simulink model "DCMG_6unit"  (R2018a)
settings: Solver=VariableStepAuto  StartTime=0.0  StopTime=3  FixedStep=0.1e-3  RelTol=1e-3
undefined symbols (not defined in the file): ALPHA, g12, g14, g23, g24, g36, g45, g56, k_ii_1, k_ii_2, k_ii_3, k_ii_4, k_ii_5, k_ii_6, k_iv_1, k_iv_2, k_iv_3, k_iv_4, k_iv_5, k_iv_6, k_pi_1, k_pi_2, k_pi_3, k_pi_4, k_pi_5, k_pi_6, k_pv_1, k_pv_2, k_pv_3, k_pv_4, k_pv_5, k_pv_6, n, p_fraction, p_k_sup, P_load_inf, P_load_sup, p_stairs, rd1, rd2, rd3, rd4, rd5, rd6, rs1, rs2, rs3, rs4, rs5, rs6, tau, time1, time2, time3, V_ref, Zout_den_source, Zout_num_source
libraries: fl_lib x62, nesl_utility x44, elec_lib x12, simulink x2
settings Model: Creator=Marco  LastModifiedBy=carna

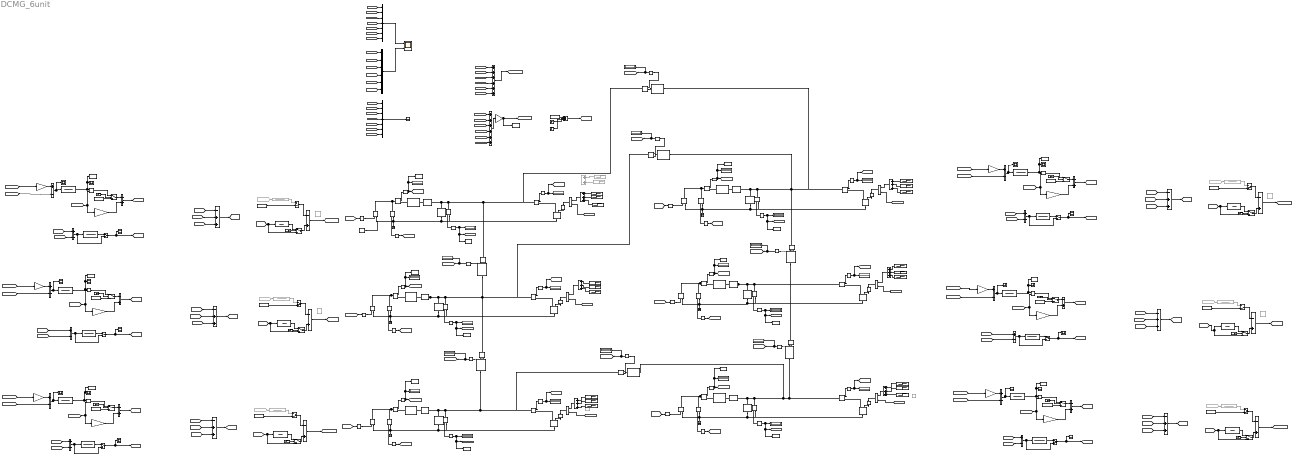
== system DCMG_6unit ==
  note: DELTA I
  note: Delta v 3
  note: I MG
  note: Delta v 1
  note: Delta R droop
  note: V MG
  note: DELTA I
  note: Delta R droop
  note: DELTA I
  note: Delta R droop
  note: Delta v 2
  note: Delta R droop
  note: Delta v 2
  note: DELTA I
  note: Delta R droop
  note: Delta R droop
  note: DELTA I
  note: Delta v 3
  note: Delta v 1
  note: DELTA I
  Add{1..2,5,7,10,12,22..23,25,31,36,38} (12 alike) : Sum  Inputs=+-
  Add{4,6,9,11,13,17,24,26,28,35,37,40} (12 alike) : Sum  Inputs=-+
  Add{3,8,14,27,34,39} (6 alike) : Sum  Inputs=-++
  Add15 : Sum  Inputs=++++++
  Add16 : Sum  Inputs=++++++
  Add{18,20..21,29,32..33,46} (7 alike) : Sum  Inputs=+++
  Add19 : Sum  Commented=on
  C bus 1 : elec_lib/Passive Devices/Capacitor  enable_table=0  c=C1 F  Cvec=[1.0e-5, 1.0e-6] F  Vvec=[0.0, 10.0] V  CV_table_symmetry=1  C_tol=5  enable_C_tol=0  tol_distribution=1  nSigma=4  r=1e-6 Ohm  g=0 1/Ohm  enable_operating_limits=0  operating_limit_action=2  max_working_voltage_range=[-25.0, 25.0] V  power_rating=1 W  enable_faults=0  fault_action=1  Cscale_faulted=100  R_faulted=1e-3 Ohm  G_faulted=0 1/Ohm  tau_fault=1e-3 s  enable_temporal_fault=0  t_fault=1 s  enable_behavioral_fault=0  max_permissible_voltage_range=[-100.0, 100.0] V  t_fail_on_voltage=1 s  i_specify=off  i_priority=None  i=0 A  i_nominal_specify=off  i_nominal_unit=A  i_nominal_value=1  v_specify=off  v_priority=None  v=0 V  v_nominal_specify=off  v_nominal_unit=V  v_nominal_value=1  vc_specify=off  vc_priority=High  vc=0 V  vc_nominal_specify=off  vc_nominal_unit=V  vc_nominal_value=1
  C bus 2 : elec_lib/Passive Devices/Capacitor  enable_table=0  c=C2 F  Cvec=[1.0e-5, 1.0e-6] F  Vvec=[0.0, 10.0] V  CV_table_symmetry=1  C_tol=5  enable_C_tol=0  tol_distribution=1  nSigma=4  r=1e-6 Ohm  g=0 1/Ohm  enable_operating_limits=0  operating_limit_action=2  max_working_voltage_range=[-25.0, 25.0] V  power_rating=1 W  enable_faults=0  fault_action=1  Cscale_faulted=100  R_faulted=1e-3 Ohm  G_faulted=0 1/Ohm  tau_fault=1e-3 s  enable_temporal_fault=0  t_fault=1 s  enable_behavioral_fault=0  max_permissible_voltage_range=[-100.0, 100.0] V  t_fail_on_voltage=1 s  i_specify=off  i_priority=None  i=0 A  i_nominal_specify=off  i_nominal_unit=A  i_nominal_value=1  v_specify=off  v_priority=None  v=0 V  v_nominal_specify=off  v_nominal_unit=V  v_nominal_value=1  vc_specify=off  vc_priority=High  vc=0 V  vc_nominal_specify=off  vc_nominal_unit=V  vc_nominal_value=1
  C bus 3 : elec_lib/Passive Devices/Capacitor  enable_table=0  c=C3 F  Cvec=[1.0e-5, 1.0e-6] F  Vvec=[0.0, 10.0] V  CV_table_symmetry=1  C_tol=5  enable_C_tol=0  tol_distribution=1  nSigma=4  r=1e-6 Ohm  g=0 1/Ohm  enable_operating_limits=0  operating_limit_action=2  max_working_voltage_range=[-25.0, 25.0] V  power_rating=1 W  enable_faults=0  fault_action=1  Cscale_faulted=100  R_faulted=1e-3 Ohm  G_faulted=0 1/Ohm  tau_fault=1e-3 s  enable_temporal_fault=0  t_fault=1 s  enable_behavioral_fault=0  max_permissible_voltage_range=[-100.0, 100.0] V  t_fail_on_voltage=1 s  i_specify=off  i_priority=None  i=0 A  i_nominal_specify=off  i_nominal_unit=A  i_nominal_value=1  v_specify=off  v_priority=None  v=0 V  v_nominal_specify=off  v_nominal_unit=V  v_nominal_value=1  vc_specify=off  vc_priority=High  vc=0 V  vc_nominal_specify=off  vc_nominal_unit=V  vc_nominal_value=1
  C bus 4 : elec_lib/Passive Devices/Capacitor  enable_table=0  c=C4 F  Cvec=[1.0e-5, 1.0e-6] F  Vvec=[0.0, 10.0] V  CV_table_symmetry=1  C_tol=5  enable_C_tol=0  tol_distribution=1  nSigma=4  r=1e-6 Ohm  g=0 1/Ohm  enable_operating_limits=0  operating_limit_action=2  max_working_voltage_range=[-25.0, 25.0] V  power_rating=1 W  enable_faults=0  fault_action=1  Cscale_faulted=100  R_faulted=1e-3 Ohm  G_faulted=0 1/Ohm  tau_fault=1e-3 s  enable_temporal_fault=0  t_fault=1 s  enable_behavioral_fault=0  max_permissible_voltage_range=[-100.0, 100.0] V  t_fail_on_voltage=1 s  i_specify=off  i_priority=None  i=0 A  i_nominal_specify=off  i_nominal_unit=A  i_nominal_value=1  v_specify=off  v_priority=None  v=0 V  v_nominal_specify=off  v_nominal_unit=V  v_nominal_value=1  vc_specify=off  vc_priority=High  vc=0 V  vc_nominal_specify=off  vc_nominal_unit=V  vc_nominal_value=1
  C bus 5 : elec_lib/Passive Devices/Capacitor  enable_table=0  c=C5 F  Cvec=[1.0e-5, 1.0e-6] F  Vvec=[0.0, 10.0] V  CV_table_symmetry=1  C_tol=5  enable_C_tol=0  tol_distribution=1  nSigma=4  r=1e-6 Ohm  g=0 1/Ohm  enable_operating_limits=0  operating_limit_action=2  max_working_voltage_range=[-25.0, 25.0] V  power_rating=1 W  enable_faults=0  fault_action=1  Cscale_faulted=100  R_faulted=1e-3 Ohm  G_faulted=0 1/Ohm  tau_fault=1e-3 s  enable_temporal_fault=0  t_fault=1 s  enable_behavioral_fault=0  max_permissible_voltage_range=[-100.0, 100.0] V  t_fail_on_voltage=1 s  i_specify=off  i_priority=None  i=0 A  i_nominal_specify=off  i_nominal_unit=A  i_nominal_value=1  v_specify=off  v_priority=None  v=0 V  v_nominal_specify=off  v_nominal_unit=V  v_nominal_value=1  vc_specify=off  vc_priority=High  vc=0 V  vc_nominal_specify=off  vc_nominal_unit=V  vc_nominal_value=1
  C bus 6 : elec_lib/Passive Devices/Capacitor  enable_table=0  c=C6 F  Cvec=[1.0e-5, 1.0e-6] F  Vvec=[0.0, 10.0] V  CV_table_symmetry=1  C_tol=5  enable_C_tol=0  tol_distribution=1  nSigma=4  r=1e-6 Ohm  g=0 1/Ohm  enable_operating_limits=0  operating_limit_action=2  max_working_voltage_range=[-25.0, 25.0] V  power_rating=1 W  enable_faults=0  fault_action=1  Cscale_faulted=100  R_faulted=1e-3 Ohm  G_faulted=0 1/Ohm  tau_fault=1e-3 s  enable_temporal_fault=0  t_fault=1 s  enable_behavioral_fault=0  max_permissible_voltage_range=[-100.0, 100.0] V  t_fail_on_voltage=1 s  i_specify=off  i_priority=None  i=0 A  i_nominal_specify=off  i_nominal_unit=A  i_nominal_value=1  v_specify=off  v_priority=None  v=0 V  v_nominal_specify=off  v_nominal_unit=V  v_nominal_value=1  vc_specify=off  vc_priority=High  vc=0 V  vc_nominal_specify=off  vc_nominal_unit=V  vc_nominal_value=1
  Close loop equivalent1 : TransferFcn  Numerator=[k_pv_1 k_iv_1 ]  Denominator=[1 0]
  Close loop equivalent{2,9..12,18} (6 alike) : TransferFcn  Numerator=[1 ]  Denominator=[tau 1]
  Close loop equivalent13 : TransferFcn  Numerator=[k_pv_5 k_iv_5 ]  Denominator=[1 0]
  Close loop equivalent{4,6,8,14..15,17} (6 alike) : TransferFcn  Commented=on  Numerator=Zout_num_source  Denominator=Zout_den_source
  Close loop equivalent16 : TransferFcn  Numerator=[k_pv_6 k_iv_6 ]  Denominator=[1 0]
  Close loop equivalent3 : TransferFcn  Numerator=[k_pv_2 k_iv_2 ]  Denominator=[1 0]
  Close loop equivalent5 : TransferFcn  Numerator=[k_pv_4 k_iv_4 ]  Denominator=[1 0]
  Close loop equivalent7 : TransferFcn  Numerator=[k_pv_3 k_iv_3 ]  Denominator=[1 0]
  Constant{1..3,5..10,15..16,18} (12 alike) : Constant  Value=0
  Constant4 : Constant  Value=V_ref
  Controlled Current Source{1..3,5..7} (6 alike) : fl_lib/Electrical/Electrical Sources/Controlled Current Source
  Controlled Voltage Source{,1..5} (6 alike) : fl_lib/Electrical/Electrical Sources/Controlled Voltage Source
  Current cloop transfer- Transport Delay{1..4} (4 alike) : TransportDelay  Commented=on  DelayTime=0.1e-3
  Current load {1..6} (6 alike) : fl_lib/Electrical/Electrical Sensors/Current Sensor
  Current output {1..13} (13 alike) : fl_lib/Electrical/Electrical Sensors/Current Sensor
  Display{,1..24} (25 alike) : Display
  Divide{1..6} (6 alike) : Product  Inputs=*/
  Electrical Reference{,1..5} (6 alike) : fl_lib/Electrical/Electrical Elements/Electrical Reference
  From17 : From  Commented=on  GotoTag=io_source_2
  From26 : From  Commented=on  GotoTag=io_source_1
  From29 : From  Commented=on  GotoTag=io_source_3
  From56 : From  Commented=on  GotoTag=io_source_2
  From63 : From  Commented=on  GotoTag=io_source_1
  From65 : From  Commented=on  GotoTag=io_source_3
  Gain1 : Gain  Gain=ALPHA(1,1)
  Gain10 : Gain  Gain=ALPHA(5,5)
  Gain11 : Gain  Gain=rd5
  Gain12 : Gain  Gain=ALPHA(6,6)
  Gain13 : Gain  Gain=rd6
  Gain2 : Gain  Gain=rd1
  Gain3 : Gain  Gain=ALPHA(2,2)
  Gain4 : Gain  Gain=rd2
  Gain5 : Gain  Gain=1/n
  Gain6 : Gain  Gain=ALPHA(3,3)
  Gain7 : Gain  Gain=rd3
  Gain8 : Gain  Gain=ALPHA(4,4)
  Gain9 : Gain  Gain=rd4
  L serie 1 : elec_lib/Passive Devices/Inductor  l=L1 H  L_tol=5  enable_L_tol=0  tol_distribution=1  nSigma=4  r=0 Ohm  g=1e-9 1/Ohm  enable_operating_limits=0  operating_limit_action=2  max_working_current=1 A  power_rating=1 W  enable_faults=0  fault_action=1  lambdaPercent=50  k_faulted=0.9999  turnsShort=0  openCct=0  groundShort=0  groundShortG=0 1/Ohm  tau_fault=1e-3 s  enable_temporal_fault=0  t_fault=1 s  enable_behavioral_fault=0  max_permissible_voltage=100 V  n_fail_on_voltage=1  max_permissible_current=1 A  t_fail_on_current=1 s  i_L_specify=off  i_L_priority=High  i_L=0 A  i_L_nominal_specify=off  i_L_nominal_unit=A  i_L_nominal_value=1
      settings: SourceProductName=Simscape Electronics  SourceProductBaseCode=SN
  L serie 2 : elec_lib/Passive Devices/Inductor  l=L2 H  L_tol=20  enable_L_tol=0  tol_distribution=1  nSigma=4  r=0 Ohm  g=1e-9 1/Ohm  enable_operating_limits=0  operating_limit_action=2  max_working_current=1 A  power_rating=1 W  enable_faults=0  fault_action=1  lambdaPercent=50  k_faulted=0.9999  turnsShort=0  openCct=0  groundShort=0  groundShortG=0 1/Ohm  tau_fault=1e-3 s  enable_temporal_fault=0  t_fault=1 s  enable_behavioral_fault=0  max_permissible_voltage=100 V  n_fail_on_voltage=1  max_permissible_current=1 A  t_fail_on_current=1 s  i_L_specify=off  i_L_priority=High  i_L=0 A  i_L_nominal_specify=off  i_L_nominal_unit=A  i_L_nominal_value=1
      settings: SourceProductName=Simscape Electronics  SourceProductBaseCode=SN
  L serie 3 : elec_lib/Passive Devices/Inductor  l=L3 H  L_tol=20  enable_L_tol=0  tol_distribution=1  nSigma=4  r=0 Ohm  g=1e-9 1/Ohm  enable_operating_limits=0  operating_limit_action=2  max_working_current=1 A  power_rating=1 W  enable_faults=0  fault_action=1  lambdaPercent=50  k_faulted=0.9999  turnsShort=0  openCct=0  groundShort=0  groundShortG=0 1/Ohm  tau_fault=1e-3 s  enable_temporal_fault=0  t_fault=1 s  enable_behavioral_fault=0  max_permissible_voltage=100 V  n_fail_on_voltage=1  max_permissible_current=1 A  t_fail_on_current=1 s  i_L_specify=off  i_L_priority=High  i_L=0 A  i_L_nominal_specify=off  i_L_nominal_unit=A  i_L_nominal_value=1
      settings: SourceProductName=Simscape Electronics  SourceProductBaseCode=SN
  L serie 4 : elec_lib/Passive Devices/Inductor  l=L4 H  L_tol=20  enable_L_tol=0  tol_distribution=1  nSigma=4  r=0 Ohm  g=1e-9 1/Ohm  enable_operating_limits=0  operating_limit_action=2  max_working_current=1 A  power_rating=1 W  enable_faults=0  fault_action=1  lambdaPercent=50  k_faulted=0.9999  turnsShort=0  openCct=0  groundShort=0  groundShortG=0 1/Ohm  tau_fault=1e-3 s  enable_temporal_fault=0  t_fault=1 s  enable_behavioral_fault=0  max_permissible_voltage=100 V  n_fail_on_voltage=1  max_permissible_current=1 A  t_fail_on_current=1 s  i_L_specify=off  i_L_priority=High  i_L=0 A  i_L_nominal_specify=off  i_L_nominal_unit=A  i_L_nominal_value=1
      settings: SourceProductName=Simscape Electronics  SourceProductBaseCode=SN
  L serie 5 : elec_lib/Passive Devices/Inductor  l=L5 H  L_tol=20  enable_L_tol=0  tol_distribution=1  nSigma=4  r=0 Ohm  g=1e-9 1/Ohm  enable_operating_limits=0  operating_limit_action=2  max_working_current=1 A  power_rating=1 W  enable_faults=0  fault_action=1  lambdaPercent=50  k_faulted=0.9999  turnsShort=0  openCct=0  groundShort=0  groundShortG=0 1/Ohm  tau_fault=1e-3 s  enable_temporal_fault=0  t_fault=1 s  enable_behavioral_fault=0  max_permissible_voltage=100 V  n_fail_on_voltage=1  max_permissible_current=1 A  t_fail_on_current=1 s  i_L_specify=off  i_L_priority=High  i_L=0 A  i_L_nominal_specify=off  i_L_nominal_unit=A  i_L_nominal_value=1
      settings: SourceProductName=Simscape Electronics  SourceProductBaseCode=SN
  L serie 6 : elec_lib/Passive Devices/Inductor  l=L6 H  L_tol=20  enable_L_tol=0  tol_distribution=1  nSigma=4  r=0 Ohm  g=1e-9 1/Ohm  enable_operating_limits=0  operating_limit_action=2  max_working_current=1 A  power_rating=1 W  enable_faults=0  fault_action=1  lambdaPercent=50  k_faulted=0.9999  turnsShort=0  openCct=0  groundShort=0  groundShortG=0 1/Ohm  tau_fault=1e-3 s  enable_temporal_fault=0  t_fault=1 s  enable_behavioral_fault=0  max_permissible_voltage=100 V  n_fail_on_voltage=1  max_permissible_current=1 A  t_fail_on_current=1 s  i_L_specify=off  i_L_priority=High  i_L=0 A  i_L_nominal_specify=off  i_L_nominal_unit=A  i_L_nominal_value=1
      settings: SourceProductName=Simscape Electronics  SourceProductBaseCode=SN
  Manual Switch{1,3,5,7,9,12} (6 alike) : ManualSwitch
  Manual Switch{2,4,6,8,10..11} (6 alike) : ManualSwitch  CurrentSetting=0
  Mux : Mux  Inputs=6
  Mux1 : Mux  Inputs=7
  Mux2 : Mux  Inputs=7
  PI i : TransferFcn  Numerator=[k_pi_1 k_ii_1 ]  Denominator=[1 0]
  PI i 1 : TransferFcn  Numerator=[k_pi_5 k_ii_5 ]  Denominator=[1 0]
  PI i 2 : TransferFcn  Numerator=[k_pi_2 k_ii_2 ]  Denominator=[1 0]
  PI i1 : TransferFcn  Numerator=[k_pi_4 k_ii_4 ]  Denominator=[1 0]
  PI i2 : TransferFcn  Numerator=[k_pi_3 k_ii_3 ]  Denominator=[1 0]
  PI i3 : TransferFcn  Numerator=[k_pi_6 k_ii_6 ]  Denominator=[1 0]
  PS-Simulink Converter{,1..30} (31 alike) : nesl_utility/PS-Simulink Converter  PhysicalDomain=network_engine_domain  SubClassName=ps_output  LeftPortType=input  RightPortType=output  PseudoPeriodic=off  Frequencies=[]  Unit=1  AffineConversion=off
  Product{,1..4,7} (6 alike) : Product
  R serie 1 : fl_lib/Electrical/Electrical Elements/Resistor  R=rs1 Ohm  i_specify=off  i_priority=None  i=0 A  i_nominal_specify=off  i_nominal_unit=A  i_nominal_value=1  v_specify=off  v_priority=None  v=0 V  v_nominal_specify=off  v_nominal_unit=V  v_nominal_value=1
  R serie 10 : fl_lib/Electrical/Electrical Elements/Resistor  R=1/g24 Ohm  i_specify=off  i_priority=None  i=0 A  i_nominal_specify=off  i_nominal_unit=A  i_nominal_value=1  v_specify=off  v_priority=None  v=0 V  v_nominal_specify=off  v_nominal_unit=V  v_nominal_value=1
  R serie 11 : fl_lib/Electrical/Electrical Elements/Resistor  R=1/g14 Ohm  i_specify=off  i_priority=None  i=0 A  i_nominal_specify=off  i_nominal_unit=A  i_nominal_value=1  v_specify=off  v_priority=None  v=0 V  v_nominal_specify=off  v_nominal_unit=V  v_nominal_value=1
  R serie 12 : fl_lib/Electrical/Electrical Elements/Resistor  R=1/g12 Ohm  i_specify=off  i_priority=None  i=0 A  i_nominal_specify=off  i_nominal_unit=A  i_nominal_value=1  v_specify=off  v_priority=None  v=0 V  v_nominal_specify=off  v_nominal_unit=V  v_nominal_value=1
  R serie 2 : fl_lib/Electrical/Electrical Elements/Resistor  R=rs2 Ohm  i_specify=off  i_priority=None  i=0 A  i_nominal_specify=off  i_nominal_unit=A  i_nominal_value=1  v_specify=off  v_priority=None  v=0 V  v_nominal_specify=off  v_nominal_unit=V  v_nominal_value=1
  R serie 23 : fl_lib/Electrical/Electrical Elements/Resistor  R=1/g23 Ohm  i_specify=off  i_priority=None  i=0 A  i_nominal_specify=off  i_nominal_unit=A  i_nominal_value=1  v_specify=off  v_priority=None  v=0 V  v_nominal_specify=off  v_nominal_unit=V  v_nominal_value=1
  R serie 3 : fl_lib/Electrical/Electrical Elements/Resistor  R=rs3 Ohm  i_specify=off  i_priority=None  i=0 A  i_nominal_specify=off  i_nominal_unit=A  i_nominal_value=1  v_specify=off  v_priority=None  v=0 V  v_nominal_specify=off  v_nominal_unit=V  v_nominal_value=1
  R serie 4 : fl_lib/Electrical/Electrical Elements/Resistor  R=rs4 Ohm  i_specify=off  i_priority=None  i=0 A  i_nominal_specify=off  i_nominal_unit=A  i_nominal_value=1  v_specify=off  v_priority=None  v=0 V  v_nominal_specify=off  v_nominal_unit=V  v_nominal_value=1
  R serie 5 : fl_lib/Electrical/Electrical Elements/Resistor  R=1/g45 Ohm  i_specify=off  i_priority=None  i=0 A  i_nominal_specify=off  i_nominal_unit=A  i_nominal_value=1  v_specify=off  v_priority=None  v=0 V  v_nominal_specify=off  v_nominal_unit=V  v_nominal_value=1
  R serie 6 : fl_lib/Electrical/Electrical Elements/Resistor  R=1/g36 Ohm  i_specify=off  i_priority=None  i=0 A  i_nominal_specify=off  i_nominal_unit=A  i_nominal_value=1  v_specify=off  v_priority=None  v=0 V  v_nominal_specify=off  v_nominal_unit=V  v_nominal_value=1
  R serie 7 : fl_lib/Electrical/Electrical Elements/Resistor  R=rs5 Ohm  i_specify=off  i_priority=None  i=0 A  i_nominal_specify=off  i_nominal_unit=A  i_nominal_value=1  v_specify=off  v_priority=None  v=0 V  v_nominal_specify=off  v_nominal_unit=V  v_nominal_value=1
  R serie 8 : fl_lib/Electrical/Electrical Elements/Resistor  R=1/g56 Ohm  i_specify=off  i_priority=None  i=0 A  i_nominal_specify=off  i_nominal_unit=A  i_nominal_value=1  v_specify=off  v_priority=None  v=0 V  v_nominal_specify=off  v_nominal_unit=V  v_nominal_value=1
  R serie 9 : fl_lib/Electrical/Electrical Elements/Resistor  R=rs6 Ohm  i_specify=off  i_priority=None  i=0 A  i_nominal_specify=off  i_nominal_unit=A  i_nominal_value=1  v_specify=off  v_priority=None  v=0 V  v_nominal_specify=off  v_nominal_unit=V  v_nominal_value=1
  Repeating Sequence Stair1 : simulink/Sources/Repeating Sequence Stair  Commented=on  OutValues=p_fraction(3) * p_stairs  tsamp=1  OutMin=[]  OutMax=[]  OutDataTypeStr=double  OutputDataTypeScalingMode=double  OutDataType=fixdt(0,8)  ConRadixGroup=Best Precision: Vector-wise  OutScaling=2^-12
  Repeating Sequence Stair2 : simulink/Sources/Repeating Sequence Stair  Commented=on  OutValues=p_fraction(3) * p_stairs  tsamp=1  OutMin=[]  OutMax=[]  OutDataTypeStr=double  OutputDataTypeScalingMode=double  OutDataType=fixdt(0,8)  ConRadixGroup=Best Precision: Vector-wise  OutScaling=2^-12
  Scope : Scope  NumInputPorts=2
  Scope{1..19} (19 alike) : Scope
  Simulink-PS Converter{,1..11} (12 alike) : nesl_utility/Simulink-PS Converter  PhysicalDomain=network_engine_domain  SubClassName=ps_input  LeftPortType=input  RightPortType=output  PseudoPeriodic=off  Frequencies=[]  NoiseDistribution=none  NoiseParameters=[]  Unit=1  AffineConversion=off  FilteringAndDerivatives=provide  SimscapeFilterOrder=1  InputFilterTimeConstant=0.001  UdotUserProvided=0
  Solver Configuration : nesl_utility/Solver Configuration  PhysicalDomain=network_engine_domain  SubClassName=solver  LeftPortType=input  RightPortType=generic  Tones=[]  Harmonics=[]  SimulateNoise=off  Profile=off  UseLocalSampling=off  EnableSwitchedLinearOptims=on  FrequencyDomain=off  UseCCode=off  RelTol=0.001  AbsTol=1e-06  MinStep=1e-09  ToWorkspace=off  RevertToSquareIcSolve=off  NumHomotopyIterations=100  PhasorMode=off  PhasorModeNumHarmonics=1  DoDC=off  ResidualTolerance=1e-09  UseLocalSolver=off  LocalSolverChoice=NE_BACKWARD_EULER_ADVANCER  LocalSolverSampleTime=0.001  DoFixedCost=off  MaxNonlinIter=3  MaxModeIter=2  LinearAlgebra=Sparse  EquationFormulation=NE_TIME_EF  DelaysMemoryBudget=1024  AutomaticFiltering=on  FilteringTimeConstant=0.001
  Step{1..2,10,14,20,22} (6 alike) : Step  Time=0  SampleTime=0
  Step11 : Step  Time=time3  After=-1*P_load_sup(4)  SampleTime=0
  Step{4,6,12,18,24,26} (6 alike) : Step  Time=0.5  SampleTime=0
  Step13 : Step  Time=time3  After=-1*P_load_sup(3)  SampleTime=0
  Step15 : Step  Time=time1  After=P_load_inf(1)  SampleTime=0
  Step16 : Step  Time=time3  After=-1*P_load_sup(6)  SampleTime=0
  Step17 : Step  Time=time2  After=-100  SampleTime=0
  Step19 : Step  Time=time2  After=P_load_sup(6)-P_load_inf(6)  SampleTime=0
  Step21 : Step  Time=time2  After=P_load_sup(4)-P_load_inf(4)  SampleTime=0
  Step23 : Step  Time=time1  After=P_load_inf(6)  SampleTime=0
  Step25 : Step  Time=time3  After=-1*P_load_sup(5)  SampleTime=0
  Step27 : Step  Time=time2  After=P_load_sup(5)-P_load_inf(5)  SampleTime=0
  Step29 : Step  Time=time1  After=P_load_inf(5)  SampleTime=0
  Step3 : Step  Time=time1  After=P_load_inf(4)  SampleTime=0
  Step31 : Step  Time=time2  After=P_load_sup(3)-P_load_inf(3)  SampleTime=0
  Step32 : Step  Time=time3  After=-1*P_load_sup(1)  SampleTime=0
  Step36 : Step  Time=time3  After=100  SampleTime=0
  Step37 : Step  Time=time1  After=P_load_inf(2)  SampleTime=0
  Step38 : Step  Time=time3  After=-1*P_load_sup(2)  SampleTime=0
  Step39 : Step  Time=time2  After=P_load_sup(2)-P_load_inf(2)  SampleTime=0
  Step5 : Step  Commented=on  Time=4  After=0.25e3  SampleTime=0
  Step7 : Step  Commented=on  After=p_fraction(1)*p_k_sup  SampleTime=0
  Step8 : Step  Time=time1  After=P_load_inf(3)  SampleTime=0
  Step9 : Step  Time=time2  After=P_load_sup(1)-P_load_inf(1)  SampleTime=0
  Switch{,4..6,10..11} (6 alike) : Switch  Criteria=u2 > Threshold  Threshold=0.5
  Switch{1..3,7..9} (6 alike) : Switch  Criteria=u2 > Threshold
  To Workspace : ToWorkspace  VariableName=i_1_sa  SaveFormat=Timeseries  SampleTime=-1
  To Workspace1 : ToWorkspace  VariableName=i_2_sa  SaveFormat=Timeseries  SampleTime=-1
  To Workspace10 : ToWorkspace  VariableName=i_4_sa  SaveFormat=Timeseries  SampleTime=-1
  To Workspace11 : ToWorkspace  VariableName=i_5_sa  SaveFormat=Timeseries  SampleTime=-1
  To Workspace12 : ToWorkspace  VariableName=i_6_sa  SaveFormat=Timeseries  SampleTime=-1
  To Workspace13 : ToWorkspace  VariableName=v_b4_sa  SaveFormat=Timeseries  SampleTime=-1
  To Workspace14 : ToWorkspace  VariableName=v_b5_sa  SaveFormat=Timeseries  SampleTime=-1
  To Workspace15 : ToWorkspace  VariableName=v_b6_sa  SaveFormat=Timeseries  SampleTime=-1
  To Workspace16 : ToWorkspace  VariableName=deltaR4_sa  SaveFormat=Timeseries  SampleTime=-1
  To Workspace17 : ToWorkspace  VariableName=deltaR5_sa  SaveFormat=Timeseries  SampleTime=-1
  To Workspace18 : ToWorkspace  VariableName=deltaR6_sa  SaveFormat=Timeseries  SampleTime=-1
  To Workspace2 : ToWorkspace  VariableName=i_3_sa  SaveFormat=Timeseries  SampleTime=-1
  To Workspace3 : ToWorkspace  VariableName=v_b1_sa  SaveFormat=Timeseries  SampleTime=-1
  To Workspace4 : ToWorkspace  VariableName=v_b2_sa  SaveFormat=Timeseries  SampleTime=-1
  To Workspace5 : ToWorkspace  VariableName=v_b3_sa  SaveFormat=Timeseries  SampleTime=-1
  To Workspace6 : ToWorkspace  VariableName=deltaR1_sa  SaveFormat=Timeseries  SampleTime=-1
  To Workspace7 : ToWorkspace  VariableName=deltaR2_sa  SaveFormat=Timeseries  SampleTime=-1
  To Workspace8 : ToWorkspace  VariableName=deltaR3_sa  SaveFormat=Timeseries  SampleTime=-1
  To Workspace9 : ToWorkspace  VariableName=V_MG_sa  SaveFormat=Timeseries  SampleTime=-1
  Voltage bus {1..6} (6 alike) : fl_lib/Electrical/Electrical Sensors/Voltage Sensor
  Voltage output {1..6} (6 alike) : fl_lib/Electrical/Electrical Sensors/Voltage Sensor
  wires:
  [delta_V_3] -> Add14/3
  Step37/1 -> Add18/1
  PS-Simulink Converter16/1 -> [i_cpl_3], Display3/1
  Step9/1 -> Add21/2
  [delta_I_3] -> Add14/1
  [io_source_1] -> Add2/2
  Step14/1 -> Switch3/2
  [V_ref_tot_1] -> Switch4/3, Close loop equivalent9/1
  PS-Simulink Converter2/1 -> To Workspace2/1, Display11/1, [io_source_3]
  Add18/1 -> Divide4/1
  Close loop equivalent9/1 -> Switch4/1
  Add4/1 -> [delta_I_1]
  [delta_V_2] -> Add8/3
  PS-Simulink Converter5/1 -> [i_cpl_1], Display/1
  Manual Switch10/1 -> Add11/1
  Manual Switch7/1 -> Scope8/1, [delta_V_3]
  PS-Simulink Converter/1 -> To Workspace/1, Display2/1, [io_source_1]
  Close loop equivalent10/1 -> Switch5/1
  Add10/1 -> Close loop equivalent7/1, Manual Switch7/2
  Step6/1 -> Switch4/2
  Step15/1 -> Add21/1
  Add14/1 -> [V_ref_tot_3]
  Add20/1 -> Divide5/1
  [V_ref_tot_3] -> Switch5/3, Close loop equivalent10/1
  [V_out2] -> Mux1/2
  PS-Simulink Converter13/1 -> Display8/1, To Workspace4/1, [v_bus_2]
  Step12/1 -> Switch5/2
  [v_bus_2] -> Add16/2
  Close loop equivalent2/1 -> Switch/1
  [i_cpl_3] -> Add15/3
  Gain5/1 -> [V_MG], To Workspace9/1
  Product7/1 -> Switch3/1
  Constant4/1 -> Add46/1
  Constant18/1 -> Manual Switch10/2
  Add46/1 -> [V_REF_c]
  Manual Switch2/1 -> Add6/1
  Gain2/1 -> Add4/2
  PS-Simulink Converter6/1 -> Display4/1, [i_bus_2_3]
  Add9/1 -> [delta_I_2]
  Switch3/1 -> Add17/1
  [v_bus_3] -> Divide5/2
  Step5/1 -> Add19/1
  Add11/1 -> [V_out_source_3]
  From29/1 -> Close loop equivalent8/1
  PS-Simulink Converter7/1 -> Display5/1, [i_bus_1_2]
  [V_out_source_2] -> Simulink-PS Converter9/1
  Add17/1 -> [delta_I_3]
  Add16/1 -> Gain5/1
  Add1/1 -> Close loop equivalent1/1, Manual Switch5/2
  [v_bus_3] -> Add16/3
  [io_source_3] -> Mux/3
  [i_cpl_1] -> Add15/1
  [i_cpl_2] -> Add15/2
  [delta_I_2] -> Add8/1
  Gain7/1 -> Add17/2
  Close loop equivalent7/1 -> Manual Switch7/1
  Constant16/1 -> Switch3/3
  Step17/1 -> Add46/2
  Add12/1 -> Scope7/1, PI i2/1
  [V_MG] -> Add10/2
  PI i 2/1 -> Product1/1, To Workspace7/1, Scope4/1
  [io_source_2] -> Product1/2, Gain4/1
  Gain6/1 -> Add12/1
  [delta_V_1] -> Add3/3
  Constant10/1 -> Switch2/3
  Switch2/1 -> Add9/1
  Step39/1 -> Add18/2
  [io_source_3] -> Add12/2
  [io_source_2] -> Add7/2
  [V_MG] -> Add5/2
  [V_REF_c] -> Add14/2
  [V_REF_c] -> Add8/2
  PI i/1 -> To Workspace6/1, Scope2/1, Product/1
  Close loop equivalent8/1 -> Manual Switch10/1
  Step4/1 -> Switch/2
  Gain3/1 -> Add7/1
  Add8/1 -> [V_ref_tot_2]
  Gain4/1 -> Add9/2
  From17/1 -> Close loop equivalent4/1
  PI i2/1 -> To Workspace8/1, Scope9/1, Product7/1
  Switch4/1 -> Add13/2
  Product1/1 -> Switch2/1
  Divide5/1 -> Simulink-PS Converter1/1
  Add2/1 -> Scope1/1, PI i/1
  [V_out1] -> Mux1/1
  Step1/1 -> Switch2/2
  Close loop equivalent3/1 -> Manual Switch1/1
  Add5/1 -> Manual Switch1/2, Close loop equivalent3/1
  [V_REF_c] -> Add3/2
  [V_REF_c] -> Add5/1
  Switch/1 -> Add6/2
  Close loop equivalent4/1 -> Manual Switch2/1
  PS-Simulink Converter3/1 -> [V_out3]
  [V_out_source_3] -> Simulink-PS Converter11/1
  [V_out3] -> Mux1/3
  [io_source_3] -> Gain7/1, Product7/2
  [V_ref_tot_2] -> Switch/3, Close loop equivalent2/1
  [v_bus_1] -> Divide3/2
  Close loop equivalent1/1 -> Manual Switch5/1
  Divide4/1 -> Simulink-PS Converter10/1
  [v_bus_2] -> Divide4/2
  PS-Simulink Converter12/1 -> [V_out2]
  Add7/1 -> Scope3/1, PI i 2/1
  PS-Simulink Converter15/1 -> To Workspace5/1, [v_bus_3], Display10/1
  [v_bus_1] -> Add16/1
  Switch5/1 -> Add11/2
  PS-Simulink Converter11/1 -> [io_source_2], To Workspace1/1, Display9/1
  Divide3/1 -> Simulink-PS Converter8/1
  [V_REF_c] -> Add10/1
  Manual Switch6/1 -> Add13/1
  Close loop equivalent6/1 -> Manual Switch6/1
  [delta_I_1] -> Add3/1
  Add3/1 -> [V_ref_tot_1]
  Constant15/1 -> Manual Switch6/2
  Step2/1 -> Switch1/2
  From26/1 -> Close loop equivalent6/1
  [io_source_1] -> Gain2/1, Product/2
  Constant8/1 -> Switch1/3
  [V_MG] -> Add1/2
  Add6/1 -> [V_out_source_2]
  Product/1 -> Switch1/1
  Add13/1 -> [V_out_source_1]
  [V_REF_c] -> Add1/1
  Manual Switch5/1 -> Scope5/1, [delta_V_1]
  [V_out_source_1] -> Simulink-PS Converter/1
  Mux/1 -> Scope/2
  [io_source_2] -> Mux/2
  Switch1/1 -> Add4/1
  PS-Simulink Converter14/1 -> Display7/1, [i_cpl_2]
  PS-Simulink Converter4/1 -> To Workspace3/1, [v_bus_1], Display1/1
  Add15/1 -> [i_MG]
  Add21/1 -> Divide3/1
  [io_source_1] -> Mux/1
  PS-Simulink Converter1/1 -> [V_out1]
  Constant3/1 -> Manual Switch2/2
  Manual Switch1/1 -> Scope6/1, [delta_V_2]
  Mux1/1 -> Scope/1
  Gain1/1 -> Add2/1
  Step7/1 -> Add19/2
  Gain8/1 -> Add31/1
  PS-Simulink Converter10/1 -> [V_out4]
  Constant7/1 -> Manual Switch8/2
  PS-Simulink Converter20/1 -> Display21/1, [i_cpl_5]
  Switch7/1 -> Add35/1
  Manual Switch9/1 -> Scope14/1, [delta_V_4]
  [V_REF_c] -> Add22/1
  Manual Switch3/1 -> Scope15/1, [delta_V_5]
  Add26/1 -> [V_out_source_4]
  [V_MG] -> Add22/2
  Product2/1 -> Switch7/1
  From63/1 -> Close loop equivalent15/1
  Add34/1 -> [V_ref_tot_4]
  Constant9/1 -> Switch7/3
  Close loop equivalent15/1 -> Manual Switch11/1
  [io_source_4] -> Gain9/1, Product2/2
  [delta_I_4] -> Add34/1
  Divide1/1 -> Simulink-PS Converter6/1
  [V_REF_c] -> Add23/1
  Switch11/1 -> Add24/2
  Manual Switch11/1 -> Add26/1
  Add38/1 -> Scope12/1, PI i 1/1
  PS-Simulink Converter18/1 -> [V_out5]
  PS-Simulink Converter21/1 -> To Workspace15/1, [v_bus_6], Display14/1
  [io_source_6] -> Gain13/1, Product4/2
  Add33/1 -> Divide1/1
  Divide2/1 -> Simulink-PS Converter4/1
  PS-Simulink Converter24/1 -> [V_out6]
  [V_REF_c] -> Add34/2
  [V_REF_c] -> Add36/1
  Close loop equivalent14/1 -> Manual Switch8/1
  Close loop equivalent13/1 -> Manual Switch3/1
  Add31/1 -> Scope10/1, PI i1/1
  Divide6/1 -> Simulink-PS Converter3/1
  Step10/1 -> Switch8/2
  Step22/1 -> Switch7/2
  [v_bus_4] -> Divide1/2
  Product3/1 -> Switch8/1
  From56/1 -> Close loop equivalent14/1
  Add39/1 -> [V_ref_tot_5]
  PI i3/1 -> To Workspace18/1, Scope18/1, Product4/1
  Gain11/1 -> Add40/2
  Gain10/1 -> Add38/1
  PI i1/1 -> To Workspace16/1, Scope11/1, Product2/1
  Close loop equivalent17/1 -> Manual Switch4/1
  Add37/1 -> [V_out_source_5]
  Switch8/1 -> Add40/1
  PS-Simulink Converter25/1 -> To Workspace13/1, [v_bus_4], Display13/1
  [io_source_5] -> Add38/2
  [io_source_6] -> Add25/2
  [delta_V_4] -> Add34/3
  Constant1/1 -> Switch8/3
  Gain12/1 -> Add25/1
  [V_ref_tot_5] -> Close loop equivalent12/1, Switch6/3
  [V_out_source_4] -> Simulink-PS Converter2/1
  [V_MG] -> Add36/2
  [io_source_5] -> Product3/2, Gain11/1
  Switch6/1 -> Add37/2
  [V_REF_c] -> Add27/2
  Switch10/1 -> Add26/2
  Add25/1 -> Scope16/1, PI i3/1
  [V_MG] -> Add23/2
  Constant2/1 -> Manual Switch11/2
  PS-Simulink Converter17/1 -> [io_source_5], To Workspace11/1, Display23/1
  [delta_I_5] -> Add39/1
  Close loop equivalent5/1 -> Manual Switch9/1
  Close loop equivalent16/1 -> Manual Switch12/1
  [v_bus_5] -> Divide2/2
  Gain13/1 -> Add28/2
  Constant5/1 -> Switch9/3
  Add28/1 -> [delta_I_6]
  Add22/1 -> Close loop equivalent5/1, Manual Switch9/2
  [V_out_source_5] -> Simulink-PS Converter7/1
  PS-Simulink Converter27/1 -> Display18/1, [i_bus_5_6]
  Add40/1 -> [delta_I_5]
  Add24/1 -> [V_out_source_6]
  Switch9/1 -> Add28/1
  Gain9/1 -> Add35/2
  Add23/1 -> Close loop equivalent16/1, Manual Switch12/2
  Step3/1 -> Add33/1
  Close loop equivalent11/1 -> Switch11/1
  [V_ref_tot_6] -> Switch11/3, Close loop equivalent11/1
  Step26/1 -> Switch10/2
  Add27/1 -> [V_ref_tot_6]
  Product4/1 -> Switch9/1
  Manual Switch8/1 -> Add37/1
  Manual Switch4/1 -> Add24/1
  PS-Simulink Converter9/1 -> To Workspace10/1, Display16/1, [io_source_4]
  PS-Simulink Converter28/1 -> Display19/1, [i_bus_4_6]
  Step24/1 -> Switch6/2
  Constant6/1 -> Manual Switch4/2
  Add29/1 -> Divide2/1
  Add36/1 -> Manual Switch3/2, Close loop equivalent13/1
  Step18/1 -> Switch11/2
  PS-Simulink Converter23/1 -> To Workspace12/1, Display15/1, [io_source_6]
  Add35/1 -> [delta_I_4]
  PS-Simulink Converter19/1 -> Display22/1, To Workspace14/1, [v_bus_5]
  PS-Simulink Converter26/1 -> [i_cpl_4], Display12/1
  [delta_V_5] -> Add39/3
  Close loop equivalent18/1 -> Switch10/1
  [io_source_4] -> Add31/2
  Step19/1 -> Add32/2
  Step20/1 -> Switch9/2
  [V_ref_tot_4] -> Switch10/3, Close loop equivalent18/1
  [v_bus_6] -> Divide6/2
  Manual Switch12/1 -> Scope17/1, [delta_V_6]
  [delta_I_6] -> Add27/1
  Add32/1 -> Divide6/1
  PS-Simulink Converter22/1 -> [i_cpl_6], Display17/1
  From65/1 -> Close loop equivalent17/1
  [delta_V_6] -> Add27/3
  [V_out_source_6] -> Simulink-PS Converter5/1
  Close loop equivalent12/1 -> Switch6/1
  Step21/1 -> Add33/2
  [V_REF_c] -> Add39/2
  PI i 1/1 -> Product3/1, To Workspace17/1, Scope13/1
  PS-Simulink Converter29/1 -> Display20/1, [i_bus_3_5]
  PS-Simulink Converter30/1 -> Display24/1, [i_bus_2_4]
  [v_bus_6] -> Add16/6
  [v_bus_5] -> Add16/5
  [v_bus_4] -> Add16/4
  [i_cpl_4] -> Add15/4
  [i_cpl_5] -> Add15/5
  [i_cpl_6] -> Add15/6
  [V_MG] -> Mux1/7
  [V_out6] -> Mux1/6
  [V_out5] -> Mux1/5
  [V_out4] -> Mux1/4
  [io_source_4] -> Mux/4
  [io_source_5] -> Mux/5
  [io_source_6] -> Mux/6
  [i_MG] -> Gain3/1
  [i_MG] -> Gain1/1
  [i_MG] -> Gain6/1
  [i_MG] -> Gain10/1
  [i_MG] -> Gain12/1
  [i_MG] -> Gain8/1
  Step8/1 -> Add20/1
  Step31/1 -> Add20/2
  Step13/1 -> Add20/3
  Step38/1 -> Add18/3
  Step32/1 -> Add21/3
  Step11/1 -> Add33/3
  Step36/1 -> Add46/3
  PS-Simulink Converter8/1 -> [i_bus_1_4], Display6/1
  Step29/1 -> Add29/1
  Step25/1 -> Add29/3
  Step16/1 -> Add32/3
  Step23/1 -> Add32/1
  Step27/1 -> Add29/2
  [v_bus_4] -> Mux2/4
  [v_bus_5] -> Mux2/5
  [v_bus_6] -> Mux2/6
  [V_MG] -> Mux2/7
  Mux2/1 -> Scope19/1
  [v_bus_3] -> Mux2/3
  [v_bus_1] -> Mux2/1
  [v_bus_2] -> Mux2/2
  connections:
  L serie 2/RConn1 -- Current output 13/LConn1 -- Current load 2/LConn1 -- Current output 5/LConn1 -- R serie 12/RConn1 -- Voltage bus 2/LConn1 -- C bus 2/LConn1
  R serie 23/RConn1 -- Current output 12/LConn1 -- Current load 3/LConn1 -- Voltage bus 3/LConn1 -- L serie 3/RConn1 -- C bus 3/LConn1
  C bus 1/RConn1 -- Controlled Voltage Source/RConn2 -- Solver Configuration/RConn1 -- Voltage output 1/RConn2 -- Electrical Reference/LConn1 -- Voltage bus 1/RConn2 -- Controlled Current Source5/LConn1
  Current output 3/LConn1 -- Voltage output 3/LConn1 -- Controlled Voltage Source1/LConn1
  Voltage bus 1/LConn1 -- C bus 1/LConn1 -- L serie 1/RConn1 -- Current output 6/LConn1 -- Current load 1/LConn1 -- Current output 4/LConn1
  C bus 3/RConn1 -- Controlled Current Source7/LConn1 -- Voltage bus 3/RConn2 -- Voltage output 3/RConn2 -- Electrical Reference2/LConn1 -- Controlled Voltage Source1/RConn2
  Voltage output 2/RConn2 -- Controlled Voltage Source3/RConn2 -- Electrical Reference1/LConn1 -- Voltage bus 2/RConn2 -- Controlled Current Source6/LConn1 -- C bus 2/RConn1
  Current output 2/LConn1 -- Controlled Voltage Source3/LConn1 -- Voltage output 2/LConn1
  Voltage output 1/LConn1 -- Controlled Voltage Source/LConn1 -- Current output 1/LConn1
  PS-Simulink Converter7/LConn1 -- Current output 4/RConn1
  Controlled Current Source5/RConn2 -- Current load 1/RConn2
  PS-Simulink Converter15/LConn1 -- Voltage bus 3/RConn1
  PS-Simulink Converter13/LConn1 -- Voltage bus 2/RConn1
  Current output 5/RConn2 -- R serie 23/LConn1
  R serie 3/LConn1 -- Current output 3/RConn2
  PS-Simulink Converter/LConn1 -- Current output 1/RConn1
  PS-Simulink Converter2/LConn1 -- Current output 3/RConn1
  Simulink-PS Converter1/RConn1 -- Controlled Current Source7/RConn1
  PS-Simulink Converter11/LConn1 -- Current output 2/RConn1
  R serie 1/LConn1 -- Current output 1/RConn2
  L serie 2/LConn1 -- R serie 2/RConn1
  Simulink-PS Converter9/RConn1 -- Controlled Voltage Source3/RConn1
  R serie 2/LConn1 -- Current output 2/RConn2
  Current output 4/RConn2 -- R serie 12/LConn1
  Simulink-PS Converter11/RConn1 -- Controlled Voltage Source1/RConn1
  PS-Simulink Converter3/LConn1 -- Voltage output 3/RConn1
  Controlled Current Source6/RConn2 -- Current load 2/RConn2
  Current load 2/RConn1 -- PS-Simulink Converter14/LConn1
  L serie 3/LConn1 -- R serie 3/RConn1
  Current load 3/RConn1 -- PS-Simulink Converter16/LConn1
  Simulink-PS Converter8/RConn1 -- Controlled Current Source5/RConn1
  Simulink-PS Converter/RConn1 -- Controlled Voltage Source/RConn1
  PS-Simulink Converter6/LConn1 -- Current output 5/RConn1
  L serie 1/LConn1 -- R serie 1/RConn1
  Controlled Current Source7/RConn2 -- Current load 3/RConn2
  PS-Simulink Converter12/LConn1 -- Voltage output 2/RConn1
  PS-Simulink Converter1/LConn1 -- Voltage output 1/RConn1
  PS-Simulink Converter4/LConn1 -- Voltage bus 1/RConn1
  Simulink-PS Converter10/RConn1 -- Controlled Current Source6/RConn1
  Current load 1/RConn1 -- PS-Simulink Converter5/LConn1
  C bus 4/RConn1 -- Voltage bus 4/RConn2 -- Controlled Current Source1/LConn1 -- Controlled Voltage Source2/RConn2 -- Voltage output 4/RConn2 -- Electrical Reference3/LConn1
  Voltage output 5/RConn2 -- Controlled Voltage Source5/RConn2 -- Electrical Reference4/LConn1 -- C bus 5/RConn1 -- Voltage bus 5/RConn2 -- Controlled Current Source2/LConn1
  C bus 6/RConn1 -- Controlled Current Source3/LConn1 -- Voltage bus 6/RConn2 -- Voltage output 6/RConn2 -- Electrical Reference5/LConn1 -- Controlled Voltage Source4/RConn2
  R serie 8/RConn1 -- Current load 6/LConn1 -- R serie 6/RConn1 -- Voltage bus 6/LConn1 -- L serie 6/RConn1 -- C bus 6/LConn1
  Current output 9/LConn1 -- Voltage output 6/LConn1 -- Controlled Voltage Source4/LConn1
  Voltage bus 4/LConn1 -- C bus 4/LConn1 -- L serie 4/RConn1 -- R serie 11/RConn1 -- Current load 4/LConn1 -- R serie 10/RConn1 -- Current output 10/LConn1
  L serie 5/RConn1 -- Current load 5/LConn1 -- Current output 11/LConn1 -- R serie 5/RConn1 -- Voltage bus 5/LConn1 -- C bus 5/LConn1
  Current output 8/LConn1 -- Controlled Voltage Source5/LConn1 -- Voltage output 5/LConn1
  Voltage output 4/LConn1 -- Controlled Voltage Source2/LConn1 -- Current output 7/LConn1
  Simulink-PS Converter7/RConn1 -- Controlled Voltage Source5/RConn1
  L serie 4/LConn1 -- R serie 4/RConn1
  PS-Simulink Converter9/LConn1 -- Current output 7/RConn1
  Current load 4/RConn1 -- PS-Simulink Converter26/LConn1
  Simulink-PS Converter5/RConn1 -- Controlled Voltage Source4/RConn1
  Current load 5/RConn1 -- PS-Simulink Converter20/LConn1
  Current output 10/RConn2 -- R serie 5/LConn1
  R serie 7/LConn1 -- Current output 8/RConn2
  PS-Simulink Converter23/LConn1 -- Current output 9/RConn1
  Simulink-PS Converter3/RConn1 -- Controlled Current Source3/RConn1
  Controlled Current Source2/RConn2 -- Current load 5/RConn2
  PS-Simulink Converter17/LConn1 -- Current output 8/RConn1
  Simulink-PS Converter2/RConn1 -- Controlled Voltage Source2/RConn1
  Current output 11/RConn2 -- R serie 8/LConn1
  PS-Simulink Converter28/LConn1 -- Current output 10/RConn1
  PS-Simulink Converter21/LConn1 -- Voltage bus 6/RConn1
  R serie 4/LConn1 -- Current output 7/RConn2
  R serie 9/LConn1 -- Current output 9/RConn2
  PS-Simulink Converter27/LConn1 -- Current output 11/RConn1
  L serie 6/LConn1 -- R serie 9/RConn1
  PS-Simulink Converter10/LConn1 -- Voltage output 4/RConn1
  PS-Simulink Converter19/LConn1 -- Voltage bus 5/RConn1
  PS-Simulink Converter24/LConn1 -- Voltage output 6/RConn1
  Current load 6/RConn1 -- PS-Simulink Converter22/LConn1
  L serie 5/LConn1 -- R serie 7/RConn1
  PS-Simulink Converter25/LConn1 -- Voltage bus 4/RConn1
  Controlled Current Source3/RConn2 -- Current load 6/RConn2
  Simulink-PS Converter4/RConn1 -- Controlled Current Source2/RConn1
  Controlled Current Source1/RConn2 -- Current load 4/RConn2
  PS-Simulink Converter18/LConn1 -- Voltage output 5/RConn1
  Simulink-PS Converter6/RConn1 -- Controlled Current Source1/RConn1
  Current output 12/RConn2 -- R serie 6/LConn1
  PS-Simulink Converter29/LConn1 -- Current output 12/RConn1
  PS-Simulink Converter30/LConn1 -- Current output 13/RConn1
  Current output 13/RConn2 -- R serie 10/LConn1
  PS-Simulink Converter8/LConn1 -- Current output 6/RConn1
  Current output 6/RConn2 -- R serie 11/LConn1
